simulink model "RPBC5602016"  (R2016b)
settings: Solver=ode45  StartTime=0.0  StopTime=100  RelTol=1e-3  EnableMultiTasking=on
values from neighbouring files (symbols this model uses):
  A1 = 1    [setupRPBC.m]
  A2 = 0.25    [setupRPBC.m]
  A3 = 0.5    [setupRPBC.m]
  A_Matrix = [A_Matrix a]    [systemident.m]
  alpha = mean(alpha)    [systemident.m]
  b1 = 0    [setupRPBC.m]
  b2 = 0    [setupRPBC.m]
  b3 = -pi/2    (= -1.57079632679)    [setupRPBC.m]
  B_Matrix = [B_Matrix B_e]    [systemident.m]
  C = 10    [RUN.m]
  N =     [Gear Ratios.mat]
  R = mean(R)    [systemident.m]
  w1 = 2    [setupRPBC.m]
  w2 = 2    [setupRPBC.m]
  w3 = 2    [setupRPBC.m]
  Z0 = [0;0;0;0;-pi/2;0]    [setupRPBC.m]
undefined symbols (not defined in the file or in its folder): statederPUMA3
settings Model: ExtModeAutoUpdateStatusClock=off  Creator=rhanz  LastModifiedBy=R4hul
settings DataIOCC: LimitDataPoints=on  SaveFormat=Array  SignalLoggingSaveFormat=ModelDataLogs
settings OptimizationCC: ExpressionDepthLimit=2147483647  InitFltsAndDblsToZero=on  LifeSpan=inf
settings DebuggingCC: SaveWithParameterizedLinksMsg=none  UnderspecifiedInitializationDetection=Classic  MergeDetectMultiDrivingBlocksExec=none  SignalResolutionControl=TryResolveAllWithWarning  MultiTaskDSMMsg=warning  MultiTaskCondExecSysMsg=none  FcnCallInpInsideContextMsg=warning  StateNameClashWarn=warning  SFUnexpectedBacktrackingDiag=warning  SFNoUnconditionalDefaultTransitionDiag=warning  SFExecutionAtInitializationDiag=none
settings HardwareCC: ProdBitPerPointer=32  ProdBitPerSizeT=32  ProdBitPerPtrDiffT=32  ProdLargestAtomicFloat=None  ProdIntDivRoundTo=Undefined  ProdEndianess=Unspecified  ProdWordSize=32  ProdHWDeviceType=32-bit Generic
settings ModelReferenceCC: PropagateSignalLabelsOutOfModel=off
settings GRTTargetCC: TargetFcnLib=ansi_tfl_tmw.mat  TargetLangStandard=C89/C90 (ANSI)  GeneratePreprocessorConditionals=Disable all  CombineOutputUpdateFcns=off  GRTInterface=on
settings ConfigComp: CovMetricSettings=dw  CovHtmlReporting=on  CovSaveCumulativeToWorkspaceVar=on  CovSaveSingleToWorkspaceVar=on  CovExternalEMLEnable=off

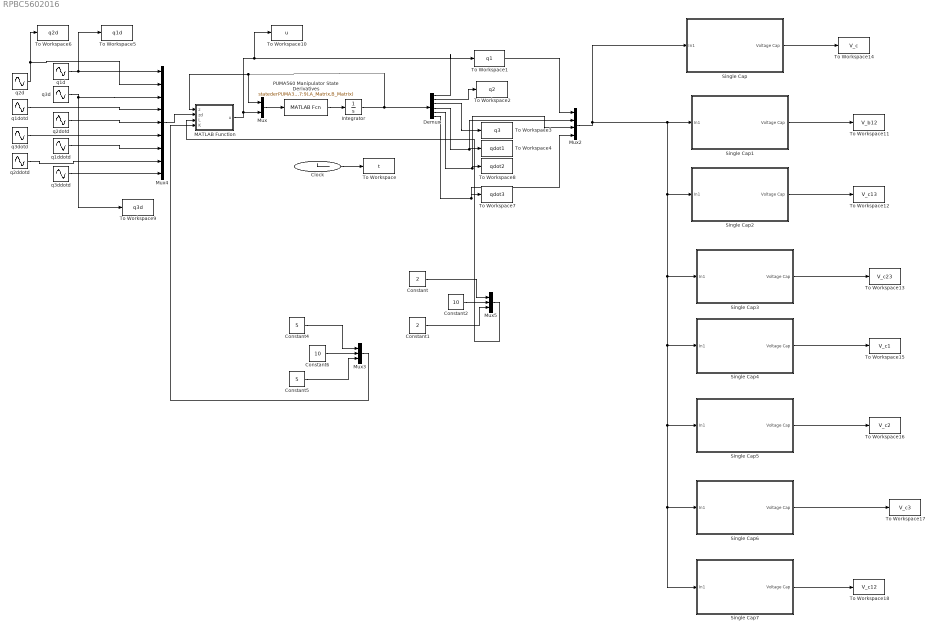
== system RPBC5602016 ==
  Clock : Clock
  Constant : Constant  Value=2
  Constant1 : Constant  Value=2
  Constant2 : Constant  Value=10
  Constant4 : Constant  Value=5
  Constant5 : Constant  Value=5
  Constant6 : Constant  Value=10
  Demux : Demux  Outputs=6
  Integrator : Integrator  InitialCondition=Z0
  MATLAB Function : MATLAB Function  TreatAsAtomicUnit=on
  Mux : Mux  Inputs=2
  Mux2 : Mux
  Mux3 : Mux  Inputs=3
  Mux4 : Mux  Inputs=9
  Mux5 : Mux  Inputs=3
  PUMA560 Manipulator State Derivatives : MATLABFcn  MATLABFcn=statederPUMA3(u(1:6),u(7:9),A_Matrix,B_Matrix)  OutputDimensions=6
  Single Cap : Subsystem
  Single Cap1 : Subsystem
  Single Cap2 : Subsystem
  Single Cap3 : Subsystem
  Single Cap4 : Subsystem
  Single Cap5 : Subsystem
  Single Cap6 : Subsystem
  Single Cap7 : Subsystem
  To Workspace : ToWorkspace  VariableName=t  SampleTime=-1
  To Workspace1 : ToWorkspace  VariableName=q1  SampleTime=-1
  To Workspace10 : ToWorkspace  VariableName=u  SampleTime=-1
  To Workspace11 : ToWorkspace  VariableName=V_b12  SampleTime=-1
  To Workspace12 : ToWorkspace  VariableName=V_c13  SampleTime=-1
  To Workspace13 : ToWorkspace  VariableName=V_c23  SampleTime=-1
  To Workspace14 : ToWorkspace  VariableName=V_c  SampleTime=-1
  To Workspace15 : ToWorkspace  VariableName=V_c1  SampleTime=-1
  To Workspace16 : ToWorkspace  VariableName=V_c2  SampleTime=-1
  To Workspace17 : ToWorkspace  VariableName=V_c3  SampleTime=-1
  To Workspace18 : ToWorkspace  VariableName=V_c12  SampleTime=-1
  To Workspace2 : ToWorkspace  VariableName=q2  SampleTime=-1
  To Workspace3 : ToWorkspace  VariableName=q3  SampleTime=-1
  To Workspace4 : ToWorkspace  VariableName=qdot1  SampleTime=-1
  To Workspace5 : ToWorkspace  VariableName=q1d  SampleTime=-1
  To Workspace6 : ToWorkspace  VariableName=q2d  SampleTime=-1
  To Workspace7 : ToWorkspace  VariableName=qdot3  SampleTime=-1
  To Workspace8 : ToWorkspace  VariableName=qdot2  SampleTime=-1
  To Workspace9 : ToWorkspace  VariableName=q3d  SampleTime=-1
  q1d : Sin  Amplitude=A1  Bias=b1  Frequency=w1  SampleTime=0
  q1ddotd : Sin  Amplitude=A1*w1^2  Frequency=w1  Phase=pi  SampleTime=0
  q1dotd : Sin  Amplitude=A1*w1  Frequency=w1  Phase=pi/2  SampleTime=0
  q2d : Sin  Amplitude=A2  Bias=b2  Frequency=w2  SampleTime=0
  q2ddotd : Sin  Amplitude=A2*w2^2  Frequency=w2  Phase=pi  SampleTime=0
  q2dotd : Sin  Amplitude=A2*w2  Frequency=w2  Phase=pi/2  SampleTime=0
  q3d : Sin  Amplitude=A3  Bias=b3  Frequency=w3  SampleTime=0
  q3ddotd : Sin  Amplitude=A3*w3^2  Frequency=w3  Phase=pi  SampleTime=0
  q3dotd : Sin  Amplitude=A3*w3  Frequency=w3  Phase=pi/2  SampleTime=0
  wires:
  PUMA560 Manipulator State Derivatives/1 -> Integrator/1
  Integrator/1 -> MATLAB Function/1(z), Mux/1, Demux/1
  Mux/1 -> PUMA560 Manipulator State Derivatives/1
  Clock/1 -> To Workspace/1
  Demux/1 -> To Workspace1/1
  Demux/3 -> To Workspace3/1
  Demux/4 -> Mux2/2, To Workspace4/1
  q1d/1 -> Mux4/1, To Workspace5/1
  q2d/1 -> Mux4/2, To Workspace6/1
  q3d/1 -> Mux4/3, To Workspace9/1
  Demux/2 -> To Workspace2/1
  Demux/5 -> Mux2/3, To Workspace8/1
  Demux/6 -> Mux2/4, To Workspace7/1
  MATLAB Function/1(u) -> Mux2/1, To Workspace10/1, Mux/2
  Single Cap/1(Voltage Cap) -> To Workspace14/1
  Mux2/1 -> Single Cap7/1(In1), Single Cap6/1(In1), Single Cap5/1(In1), Single Cap4/1(In1), Single Cap3/1(In1), Single Cap2/1(In1), Single Cap1/1(In1), Single Cap/1(In1)
  Single Cap1/1(Voltage Cap) -> To Workspace11/1
  Single Cap2/1(Voltage Cap) -> To Workspace12/1
  Single Cap3/1(Voltage Cap) -> To Workspace13/1
  Single Cap4/1(Voltage Cap) -> To Workspace15/1
  Single Cap6/1(Voltage Cap) -> To Workspace17/1
  Single Cap5/1(Voltage Cap) -> To Workspace16/1
  Single Cap7/1(Voltage Cap) -> To Workspace18/1
  Constant5/1 -> Mux3/3
  Constant6/1 -> Mux3/2
  Constant4/1 -> Mux3/1
  Mux3/1 -> MATLAB Function/4(K)
  Constant2/1 -> Mux5/2
  Constant1/1 -> Mux5/3
  Constant/1 -> Mux5/1
  Mux5/1 -> MATLAB Function/3(L)
  Mux4/1 -> MATLAB Function/2(zd)
  q1dotd/1 -> Mux4/4
  q2dotd/1 -> Mux4/5
  q3dotd/1 -> Mux4/6
  q1ddotd/1 -> Mux4/7
  q2ddotd/1 -> Mux4/8
  q3ddotd/1 -> Mux4/9

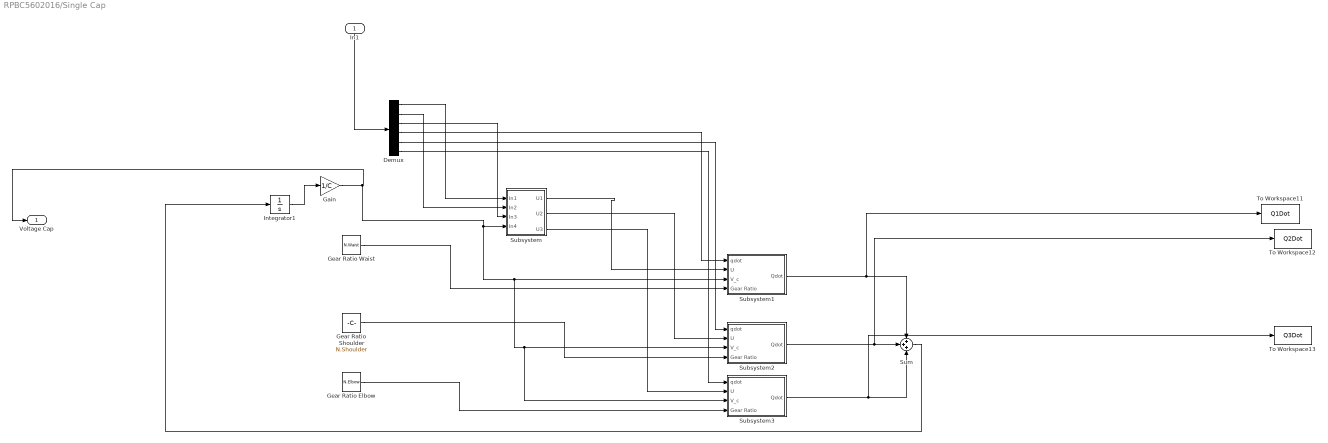
== system RPBC5602016/Single Cap ==
  In1 : Inport
  Demux : Demux  Outputs=6
  Gain : Gain  Gain=1/C
  Gear Ratio Elbow : Constant  Value=N.Elbow
  "Gear Ratio Shoulder " : Constant  Value=N.Shoulder
  Gear Ratio Waist : Constant  Value=N.Waist
  Integrator1 : Integrator  InitialCondition=C*30
  Subsystem : Subsystem
  Subsystem1 : Subsystem
  Subsystem2 : Subsystem
  Subsystem3 : Subsystem
  Sum : Sum  Inputs=3
  To Workspace11 : ToWorkspace  VariableName=Q1Dot  SampleTime=-1
  To Workspace12 : ToWorkspace  VariableName=Q2Dot  SampleTime=-1
  To Workspace13 : ToWorkspace  VariableName=Q3Dot  SampleTime=-1
  Voltage Cap : Outport
  wires:
  Subsystem/2(U2) -> Subsystem2/2(U)
  Gear Ratio Waist/1 -> Subsystem1/4(Gear Ratio)
  Subsystem/1(U1) -> Subsystem1/2(U)
  Subsystem3/1(Qdot) -> To Workspace13/1, Sum/3
  Integrator1/1 -> Gain/1
  Subsystem1/1(Qdot) -> To Workspace11/1, Sum/1
  Subsystem/3(U3) -> Subsystem3/2(U)
  Subsystem2/1(Qdot) -> To Workspace12/1, Sum/2
  Sum/1 -> Integrator1/1
  Gear Ratio Elbow/1 -> Subsystem3/4(Gear Ratio)
  "Gear Ratio Shoulder "/1 -> Subsystem2/4(Gear Ratio)
  Gain/1 -> Subsystem/4(In4), Subsystem3/3(V_c), Subsystem2/3(V_c), Subsystem1/3(V_c), Voltage Cap/1
  In1/1 -> Demux/1
  Demux/1 -> Subsystem/1(In1)
  Demux/2 -> Subsystem/2(In2)
  Demux/3 -> Subsystem/3(In3)
  Demux/4 -> Subsystem1/1(qdot)
  Demux/5 -> Subsystem2/1(qdot)
  Demux/6 -> Subsystem3/1(qdot)

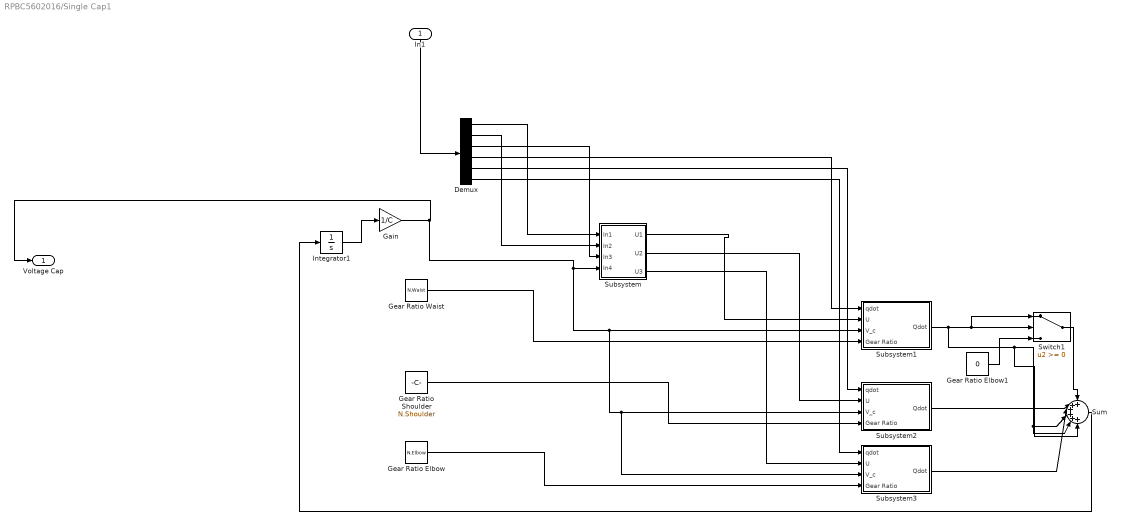
== system RPBC5602016/Single Cap1 ==
  In1 : Inport
  Demux : Demux  Outputs=6
  Gain : Gain  Gain=1/C
  Gear Ratio Elbow : Constant  Value=N.Elbow
  Gear Ratio Elbow1 : Constant  Value=0
  "Gear Ratio Shoulder " : Constant  Value=N.Shoulder
  Gear Ratio Waist : Constant  Value=N.Waist
  Integrator1 : Integrator  InitialCondition=C*30
  Subsystem : Subsystem
  Subsystem1 : Subsystem
  Subsystem2 : Subsystem
  Subsystem3 : Subsystem
  Sum : Sum  Inputs=6
  Switch1 : Switch
  Voltage Cap : Outport
  wires:
  Demux/6 -> Subsystem3/1(qdot)
  Demux/5 -> Subsystem2/1(qdot)
  Demux/4 -> Subsystem1/1(qdot)
  Demux/3 -> Subsystem/3(In3)
  Demux/2 -> Subsystem/2(In2)
  Demux/1 -> Subsystem/1(In1)
  In1/1 -> Demux/1
  Gain/1 -> Voltage Cap/1, Subsystem1/3(V_c), Subsystem2/3(V_c), Subsystem3/3(V_c), Subsystem/4(In4)
  "Gear Ratio Shoulder "/1 -> Subsystem2/4(Gear Ratio)
  Gear Ratio Elbow/1 -> Subsystem3/4(Gear Ratio)
  Subsystem2/1(Qdot) -> Sum/2
  Subsystem/3(U3) -> Subsystem3/2(U)
  Integrator1/1 -> Gain/1
  Subsystem/1(U1) -> Subsystem1/2(U)
  Gear Ratio Waist/1 -> Subsystem1/4(Gear Ratio)
  Subsystem/2(U2) -> Subsystem2/2(U)
  Subsystem3/1(Qdot) -> Sum/3
  Sum/1 -> Integrator1/1
  Subsystem1/1(Qdot) -> Sum/6, Sum/5, Sum/4, Switch1/1, Switch1/2
  Switch1/1 -> Sum/1
  Gear Ratio Elbow1/1 -> Switch1/3

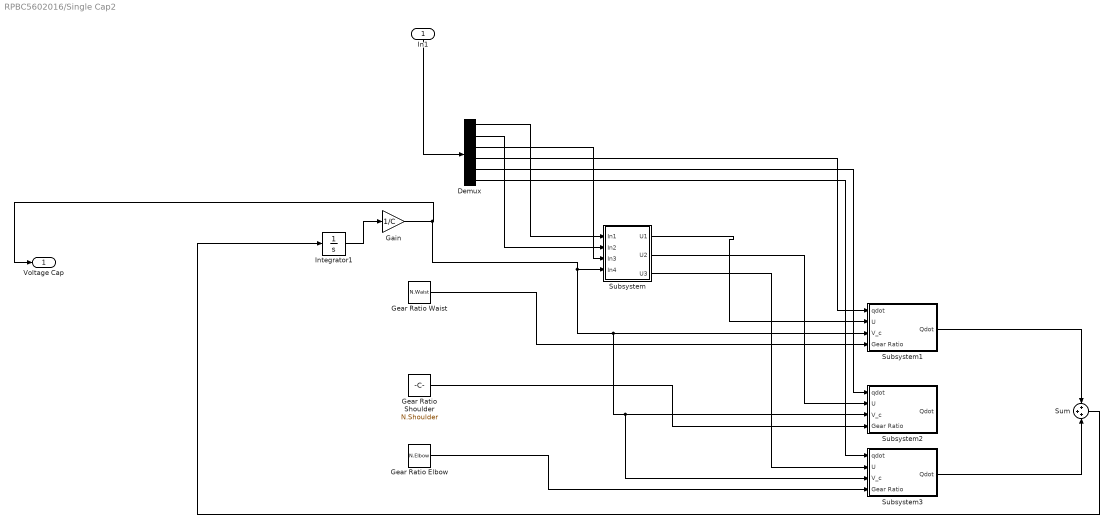
== system RPBC5602016/Single Cap2 ==
  In1 : Inport
  Demux : Demux  Outputs=6
  Gain : Gain  Gain=1/C
  Gear Ratio Elbow : Constant  Value=N.Elbow
  "Gear Ratio Shoulder " : Constant  Value=N.Shoulder
  Gear Ratio Waist : Constant  Value=N.Waist
  Integrator1 : Integrator  InitialCondition=C*30
  Subsystem : Subsystem
  Subsystem1 : Subsystem
  Subsystem2 : Subsystem
  Subsystem3 : Subsystem
  Sum : Sum  Inputs=3
  Voltage Cap : Outport
  wires:
  Subsystem/2(U2) -> Subsystem2/2(U)
  Gear Ratio Waist/1 -> Subsystem1/4(Gear Ratio)
  Subsystem/1(U1) -> Subsystem1/2(U)
  Subsystem3/1(Qdot) -> Sum/3
  Integrator1/1 -> Gain/1
  Subsystem1/1(Qdot) -> Sum/1
  Subsystem/3(U3) -> Subsystem3/2(U)
  Sum/1 -> Integrator1/1
  Gear Ratio Elbow/1 -> Subsystem3/4(Gear Ratio)
  "Gear Ratio Shoulder "/1 -> Subsystem2/4(Gear Ratio)
  Gain/1 -> Subsystem/4(In4), Subsystem3/3(V_c), Subsystem2/3(V_c), Subsystem1/3(V_c), Voltage Cap/1
  In1/1 -> Demux/1
  Demux/1 -> Subsystem/1(In1)
  Demux/2 -> Subsystem/2(In2)
  Demux/3 -> Subsystem/3(In3)
  Demux/4 -> Subsystem1/1(qdot)
  Demux/5 -> Subsystem2/1(qdot)
  Demux/6 -> Subsystem3/1(qdot)

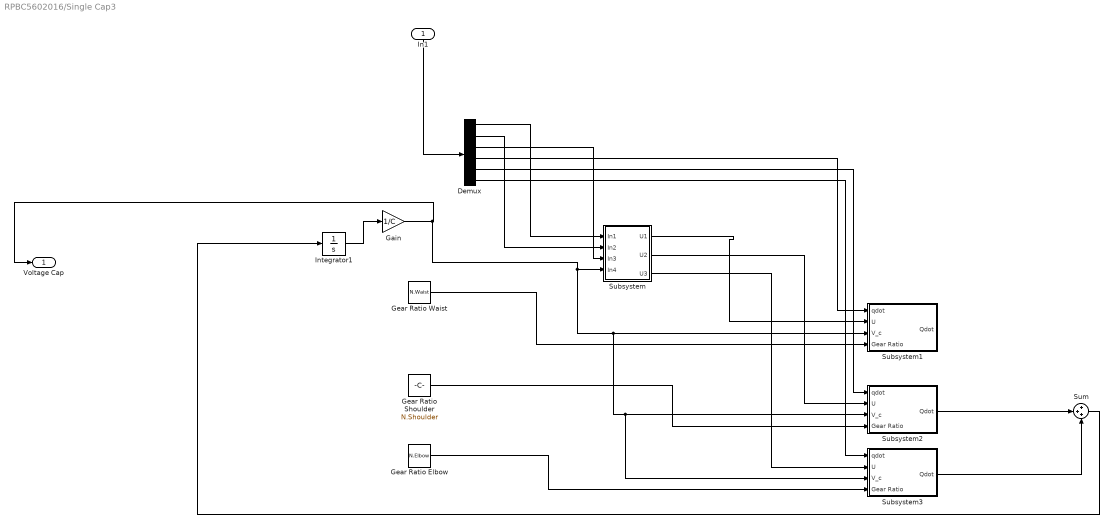
== system RPBC5602016/Single Cap3 ==
  In1 : Inport
  Demux : Demux  Outputs=6
  Gain : Gain  Gain=1/C
  Gear Ratio Elbow : Constant  Value=N.Elbow
  "Gear Ratio Shoulder " : Constant  Value=N.Shoulder
  Gear Ratio Waist : Constant  Value=N.Waist
  Integrator1 : Integrator  InitialCondition=C*30
  Subsystem : Subsystem
  Subsystem1 : Subsystem
  Subsystem2 : Subsystem
  Subsystem3 : Subsystem
  Sum : Sum  Inputs=3
  Voltage Cap : Outport
  wires:
  Demux/6 -> Subsystem3/1(qdot)
  Demux/5 -> Subsystem2/1(qdot)
  Demux/4 -> Subsystem1/1(qdot)
  Demux/3 -> Subsystem/3(In3)
  Demux/2 -> Subsystem/2(In2)
  Demux/1 -> Subsystem/1(In1)
  In1/1 -> Demux/1
  Gain/1 -> Voltage Cap/1, Subsystem1/3(V_c), Subsystem2/3(V_c), Subsystem3/3(V_c), Subsystem/4(In4)
  "Gear Ratio Shoulder "/1 -> Subsystem2/4(Gear Ratio)
  Gear Ratio Elbow/1 -> Subsystem3/4(Gear Ratio)
  Sum/1 -> Integrator1/1
  Subsystem2/1(Qdot) -> Sum/2
  Subsystem/3(U3) -> Subsystem3/2(U)
  Integrator1/1 -> Gain/1
  Subsystem3/1(Qdot) -> Sum/3
  Subsystem/1(U1) -> Subsystem1/2(U)
  Gear Ratio Waist/1 -> Subsystem1/4(Gear Ratio)
  Subsystem/2(U2) -> Subsystem2/2(U)

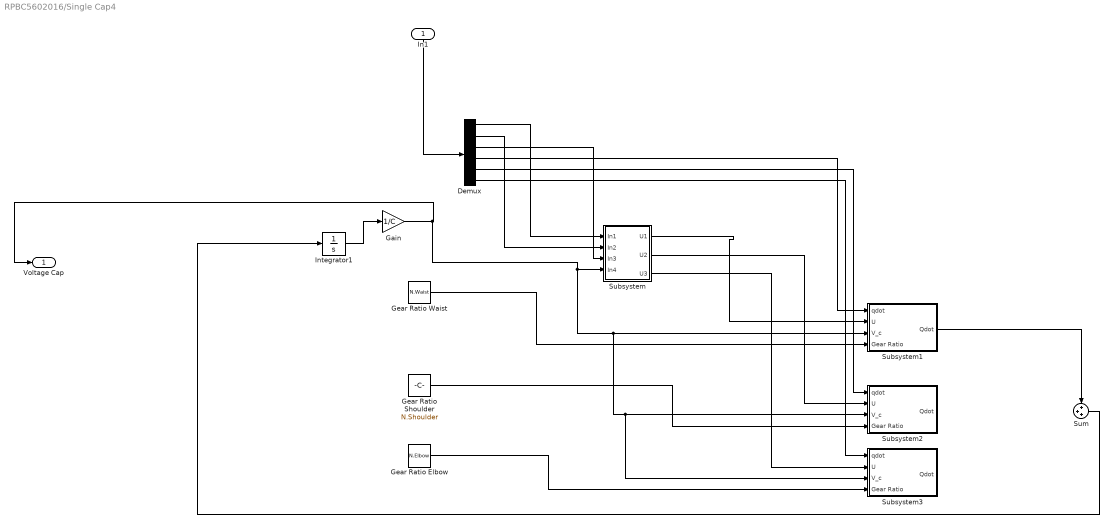
== system RPBC5602016/Single Cap4 ==
  In1 : Inport
  Demux : Demux  Outputs=6
  Gain : Gain  Gain=1/C
  Gear Ratio Elbow : Constant  Value=N.Elbow
  "Gear Ratio Shoulder " : Constant  Value=N.Shoulder
  Gear Ratio Waist : Constant  Value=N.Waist
  Integrator1 : Integrator  InitialCondition=C*30
  Subsystem : Subsystem
  Subsystem1 : Subsystem
  Subsystem2 : Subsystem
  Subsystem3 : Subsystem
  Sum : Sum  Inputs=3
  Voltage Cap : Outport
  wires:
  Subsystem/2(U2) -> Subsystem2/2(U)
  Gear Ratio Waist/1 -> Subsystem1/4(Gear Ratio)
  Subsystem/1(U1) -> Subsystem1/2(U)
  Integrator1/1 -> Gain/1
  Subsystem/3(U3) -> Subsystem3/2(U)
  Sum/1 -> Integrator1/1
  Gear Ratio Elbow/1 -> Subsystem3/4(Gear Ratio)
  "Gear Ratio Shoulder "/1 -> Subsystem2/4(Gear Ratio)
  Gain/1 -> Subsystem/4(In4), Subsystem3/3(V_c), Subsystem2/3(V_c), Subsystem1/3(V_c), Voltage Cap/1
  In1/1 -> Demux/1
  Demux/1 -> Subsystem/1(In1)
  Demux/2 -> Subsystem/2(In2)
  Demux/3 -> Subsystem/3(In3)
  Demux/4 -> Subsystem1/1(qdot)
  Demux/5 -> Subsystem2/1(qdot)
  Demux/6 -> Subsystem3/1(qdot)
  Subsystem1/1(Qdot) -> Sum/1

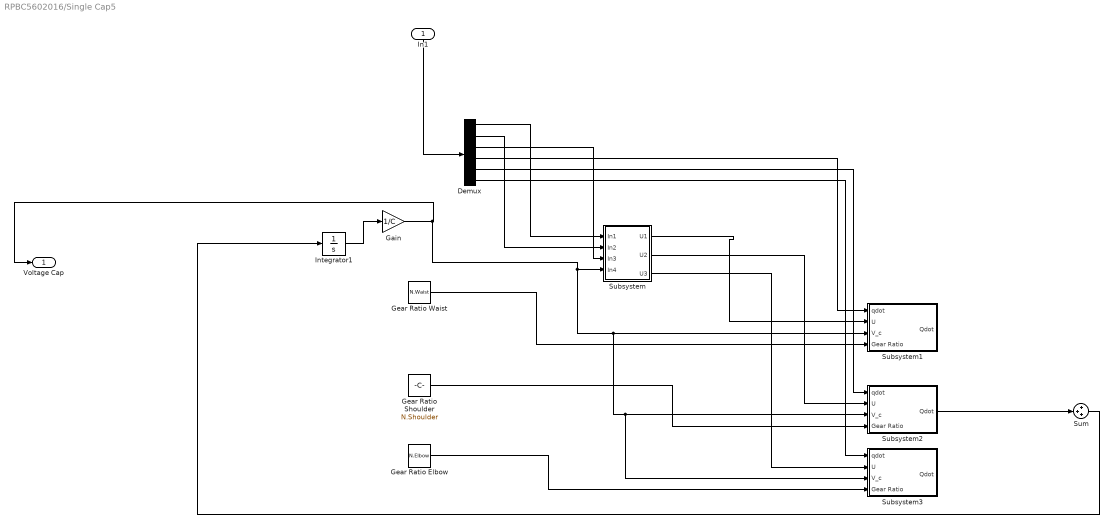
== system RPBC5602016/Single Cap5 ==
  In1 : Inport
  Demux : Demux  Outputs=6
  Gain : Gain  Gain=1/C
  Gear Ratio Elbow : Constant  Value=N.Elbow
  "Gear Ratio Shoulder " : Constant  Value=N.Shoulder
  Gear Ratio Waist : Constant  Value=N.Waist
  Integrator1 : Integrator  InitialCondition=C*30
  Subsystem : Subsystem
  Subsystem1 : Subsystem
  Subsystem2 : Subsystem
  Subsystem3 : Subsystem
  Sum : Sum  Inputs=3
  Voltage Cap : Outport
  wires:
  Demux/6 -> Subsystem3/1(qdot)
  Demux/5 -> Subsystem2/1(qdot)
  Demux/4 -> Subsystem1/1(qdot)
  Demux/3 -> Subsystem/3(In3)
  Demux/2 -> Subsystem/2(In2)
  Demux/1 -> Subsystem/1(In1)
  In1/1 -> Demux/1
  Gain/1 -> Voltage Cap/1, Subsystem1/3(V_c), Subsystem2/3(V_c), Subsystem3/3(V_c), Subsystem/4(In4)
  "Gear Ratio Shoulder "/1 -> Subsystem2/4(Gear Ratio)
  Gear Ratio Elbow/1 -> Subsystem3/4(Gear Ratio)
  Sum/1 -> Integrator1/1
  Subsystem2/1(Qdot) -> Sum/2
  Subsystem/3(U3) -> Subsystem3/2(U)
  Integrator1/1 -> Gain/1
  Subsystem/1(U1) -> Subsystem1/2(U)
  Gear Ratio Waist/1 -> Subsystem1/4(Gear Ratio)
  Subsystem/2(U2) -> Subsystem2/2(U)

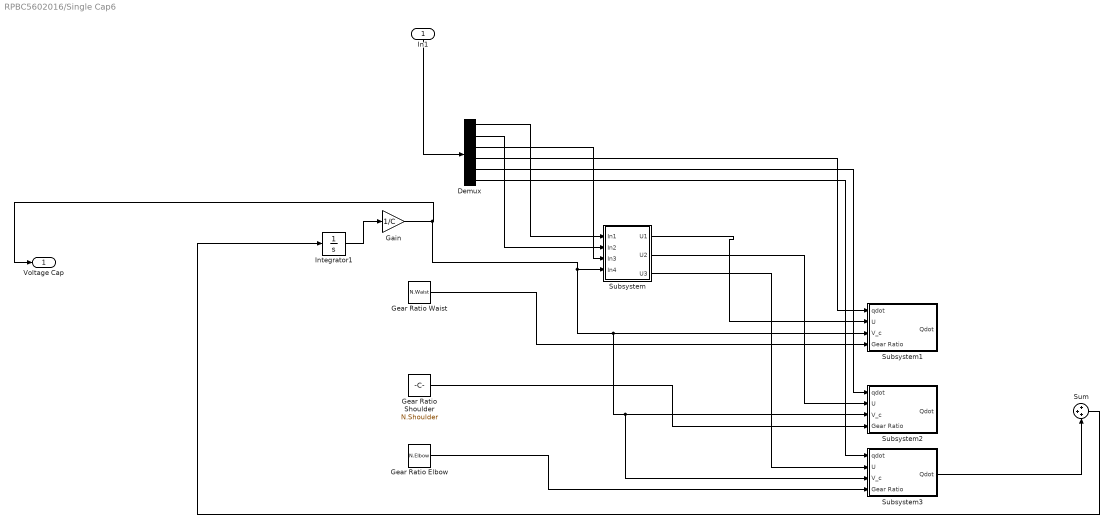
== system RPBC5602016/Single Cap6 ==
  In1 : Inport
  Demux : Demux  Outputs=6
  Gain : Gain  Gain=1/C
  Gear Ratio Elbow : Constant  Value=N.Elbow
  "Gear Ratio Shoulder " : Constant  Value=N.Shoulder
  Gear Ratio Waist : Constant  Value=N.Waist
  Integrator1 : Integrator  InitialCondition=C*30
  Subsystem : Subsystem
  Subsystem1 : Subsystem
  Subsystem2 : Subsystem
  Subsystem3 : Subsystem
  Sum : Sum  Inputs=3
  Voltage Cap : Outport
  wires:
  Subsystem/2(U2) -> Subsystem2/2(U)
  Gear Ratio Waist/1 -> Subsystem1/4(Gear Ratio)
  Subsystem/1(U1) -> Subsystem1/2(U)
  Subsystem3/1(Qdot) -> Sum/3
  Integrator1/1 -> Gain/1
  Subsystem/3(U3) -> Subsystem3/2(U)
  Sum/1 -> Integrator1/1
  Gear Ratio Elbow/1 -> Subsystem3/4(Gear Ratio)
  "Gear Ratio Shoulder "/1 -> Subsystem2/4(Gear Ratio)
  Gain/1 -> Subsystem/4(In4), Subsystem3/3(V_c), Subsystem2/3(V_c), Subsystem1/3(V_c), Voltage Cap/1
  In1/1 -> Demux/1
  Demux/1 -> Subsystem/1(In1)
  Demux/2 -> Subsystem/2(In2)
  Demux/3 -> Subsystem/3(In3)
  Demux/4 -> Subsystem1/1(qdot)
  Demux/5 -> Subsystem2/1(qdot)
  Demux/6 -> Subsystem3/1(qdot)

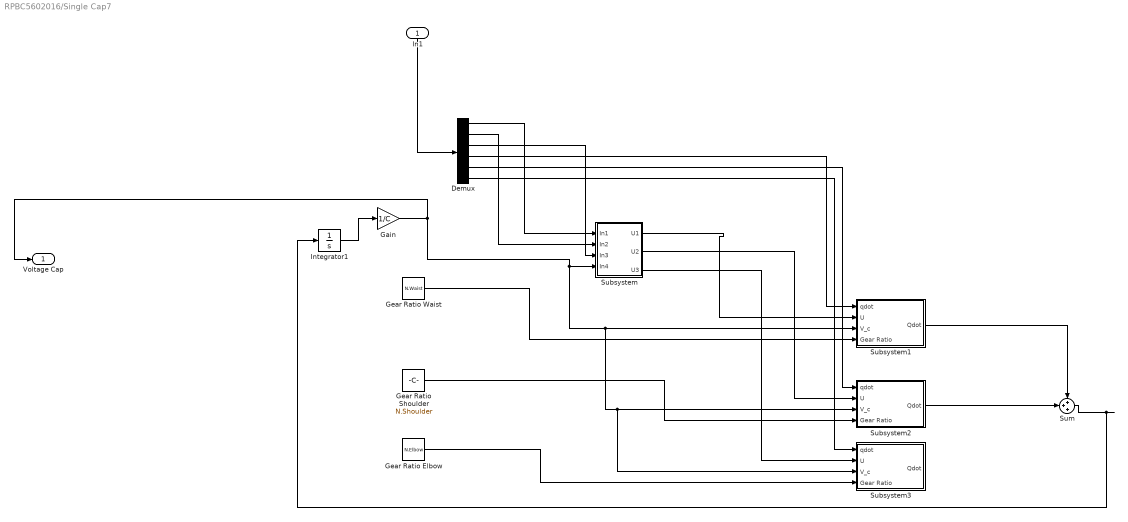
== system RPBC5602016/Single Cap7 ==
  In1 : Inport
  Demux : Demux  Outputs=6
  Gain : Gain  Gain=1/C
  Gear Ratio Elbow : Constant  Value=N.Elbow
  "Gear Ratio Shoulder " : Constant  Value=N.Shoulder
  Gear Ratio Waist : Constant  Value=N.Waist
  Integrator1 : Integrator  InitialCondition=C*30
  Subsystem : Subsystem
  Subsystem1 : Subsystem
  Subsystem2 : Subsystem
  Subsystem3 : Subsystem
  Sum : Sum  Inputs=3
  Voltage Cap : Outport
  wires:
  Sum/1 -> Integrator1/1
  Subsystem/2(U2) -> Subsystem2/2(U)
  Gear Ratio Waist/1 -> Subsystem1/4(Gear Ratio)
  Subsystem/1(U1) -> Subsystem1/2(U)
  Integrator1/1 -> Gain/1
  Subsystem1/1(Qdot) -> Sum/1
  Subsystem/3(U3) -> Subsystem3/2(U)
  Subsystem2/1(Qdot) -> Sum/2
  Gear Ratio Elbow/1 -> Subsystem3/4(Gear Ratio)
  "Gear Ratio Shoulder "/1 -> Subsystem2/4(Gear Ratio)
  Gain/1 -> Subsystem/4(In4), Subsystem3/3(V_c), Subsystem2/3(V_c), Subsystem1/3(V_c), Voltage Cap/1
  In1/1 -> Demux/1
  Demux/1 -> Subsystem/1(In1)
  Demux/2 -> Subsystem/2(In2)
  Demux/3 -> Subsystem/3(In3)
  Demux/4 -> Subsystem1/1(qdot)
  Demux/5 -> Subsystem2/1(qdot)
  Demux/6 -> Subsystem3/1(qdot)

== system RPBC5602016/Single Cap/Subsystem ==
  In1 : Inport
  In2 : Inport  Port=2
  In3 : Inport  Port=3
  In4 : Inport  Port=4
  Divide : Product  Inputs=*/
  Divide1 : Product  Inputs=*/
  Divide2 : Product  Inputs=*/
  U1 : Outport
  U2 : Outport  Port=2
  U3 : Outport  Port=3
  wires:
  Divide2/1 -> U3/1
  Divide1/1 -> U2/1
  Divide/1 -> U1/1
  In1/1 -> Divide/1
  In2/1 -> Divide1/1
  In3/1 -> Divide2/1
  In4/1 -> Divide2/2, Divide1/2, Divide/2

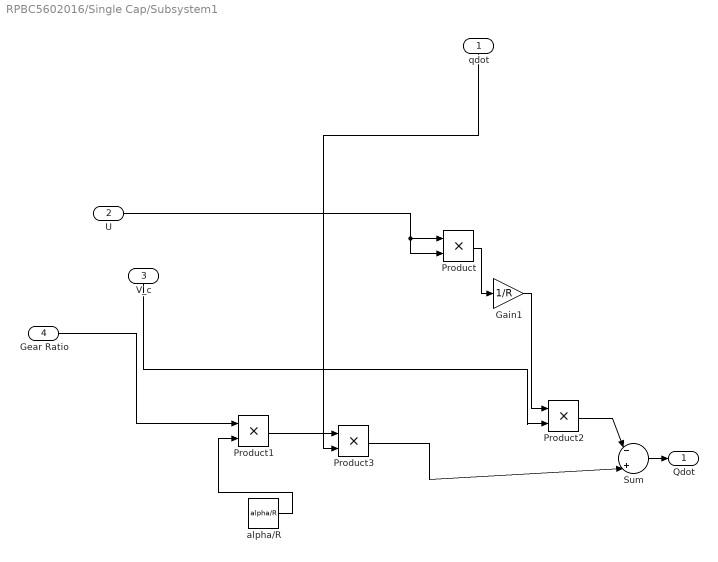
== system RPBC5602016/Single Cap/Subsystem1 ==
  qdot : Inport
  U : Inport  Port=2
  V_c : Inport  Port=3
  Gear Ratio : Inport  Port=4
  Gain1 : Gain  Gain=1/R
  Product{,1..3} (4 alike) : Product
  Sum : Sum  Inputs=|-|+|
  alpha/R : Constant  Value=alpha/R
  Qdot : Outport
  wires:
  Product2/1 -> Sum/1
  qdot/1 -> Product3/2
  V_c/1 -> Product2/2
  Sum/1 -> Qdot/1
  alpha/R/1 -> Product1/2
  Product/1 -> Gain1/1
  U/1 -> Product/2, Product/1
  Product3/1 -> Sum/2
  Product1/1 -> Product3/1
  Gain1/1 -> Product2/1
  Gear Ratio/1 -> Product1/1

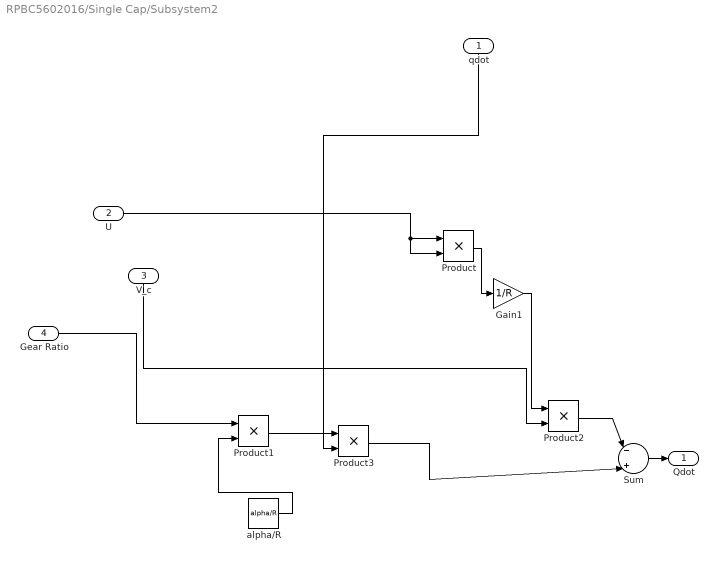
== system RPBC5602016/Single Cap/Subsystem2 ==
  qdot : Inport
  U : Inport  Port=2
  V_c : Inport  Port=3
  Gear Ratio : Inport  Port=4
  Gain1 : Gain  Gain=1/R
  Product{,1..3} (4 alike) : Product
  Sum : Sum  Inputs=|-|+|
  alpha/R : Constant  Value=alpha/R
  Qdot : Outport
  wires:
  Gear Ratio/1 -> Product1/1
  Gain1/1 -> Product2/1
  Product1/1 -> Product3/1
  Product3/1 -> Sum/2
  U/1 -> Product/1, Product/2
  Product/1 -> Gain1/1
  alpha/R/1 -> Product1/2
  Sum/1 -> Qdot/1
  V_c/1 -> Product2/2
  qdot/1 -> Product3/2
  Product2/1 -> Sum/1

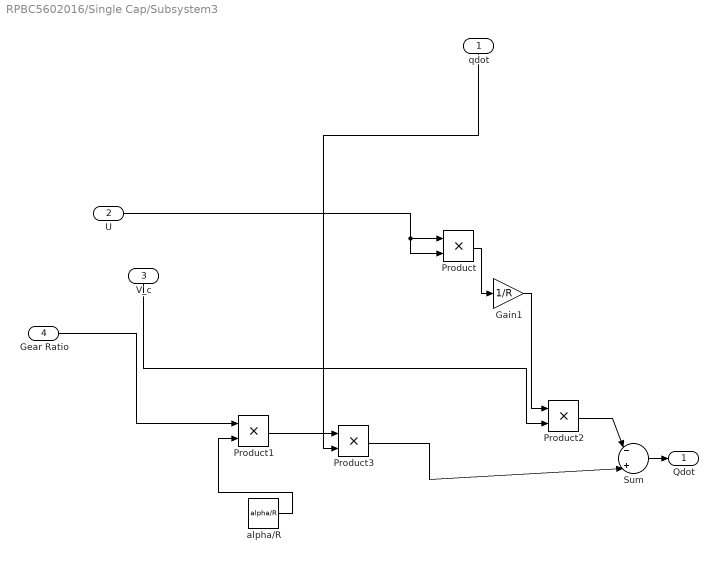
== system RPBC5602016/Single Cap/Subsystem3 ==
  qdot : Inport
  U : Inport  Port=2
  V_c : Inport  Port=3
  Gear Ratio : Inport  Port=4
  Gain1 : Gain  Gain=1/R
  Product{,1..3} (4 alike) : Product
  Sum : Sum  Inputs=|-|+|
  alpha/R : Constant  Value=alpha/R
  Qdot : Outport
  wires:
  Product2/1 -> Sum/1
  qdot/1 -> Product3/2
  V_c/1 -> Product2/2
  Sum/1 -> Qdot/1
  alpha/R/1 -> Product1/2
  Product/1 -> Gain1/1
  U/1 -> Product/2, Product/1
  Product3/1 -> Sum/2
  Product1/1 -> Product3/1
  Gain1/1 -> Product2/1
  Gear Ratio/1 -> Product1/1

== system RPBC5602016/Single Cap1/Subsystem ==
  In1 : Inport
  In2 : Inport  Port=2
  In3 : Inport  Port=3
  In4 : Inport  Port=4
  Divide : Product  Inputs=*/
  Divide1 : Product  Inputs=*/
  Divide2 : Product  Inputs=*/
  U1 : Outport
  U2 : Outport  Port=2
  U3 : Outport  Port=3
  wires:
  In4/1 -> Divide/2, Divide1/2, Divide2/2
  In3/1 -> Divide2/1
  In2/1 -> Divide1/1
  In1/1 -> Divide/1
  Divide/1 -> U1/1
  Divide1/1 -> U2/1
  Divide2/1 -> U3/1

== system RPBC5602016/Single Cap1/Subsystem1 ==
  qdot : Inport
  U : Inport  Port=2
  V_c : Inport  Port=3
  Gear Ratio : Inport  Port=4
  Gain1 : Gain  Gain=1/R
  Product{,1..3} (4 alike) : Product
  Sum : Sum  Inputs=|-|+|
  alpha/R : Constant  Value=alpha/R
  Qdot : Outport
  wires:
  Gear Ratio/1 -> Product1/1
  Gain1/1 -> Product2/1
  Product1/1 -> Product3/1
  Product3/1 -> Sum/2
  U/1 -> Product/1, Product/2
  Product/1 -> Gain1/1
  alpha/R/1 -> Product1/2
  Sum/1 -> Qdot/1
  V_c/1 -> Product2/2
  qdot/1 -> Product3/2
  Product2/1 -> Sum/1

== system RPBC5602016/Single Cap1/Subsystem2 ==
  qdot : Inport
  U : Inport  Port=2
  V_c : Inport  Port=3
  Gear Ratio : Inport  Port=4
  Gain1 : Gain  Gain=1/R
  Product{,1..3} (4 alike) : Product
  Sum : Sum  Inputs=|-|+|
  alpha/R : Constant  Value=alpha/R
  Qdot : Outport
  wires:
  Product2/1 -> Sum/1
  qdot/1 -> Product3/2
  V_c/1 -> Product2/2
  Sum/1 -> Qdot/1
  alpha/R/1 -> Product1/2
  Product/1 -> Gain1/1
  U/1 -> Product/2, Product/1
  Product3/1 -> Sum/2
  Product1/1 -> Product3/1
  Gain1/1 -> Product2/1
  Gear Ratio/1 -> Product1/1

== system RPBC5602016/Single Cap1/Subsystem3 ==
  qdot : Inport
  U : Inport  Port=2
  V_c : Inport  Port=3
  Gear Ratio : Inport  Port=4
  Gain1 : Gain  Gain=1/R
  Product{,1..3} (4 alike) : Product
  Sum : Sum  Inputs=|-|+|
  alpha/R : Constant  Value=alpha/R
  Qdot : Outport
  wires:
  Gear Ratio/1 -> Product1/1
  Gain1/1 -> Product2/1
  Product1/1 -> Product3/1
  Product3/1 -> Sum/2
  U/1 -> Product/1, Product/2
  Product/1 -> Gain1/1
  alpha/R/1 -> Product1/2
  Sum/1 -> Qdot/1
  V_c/1 -> Product2/2
  qdot/1 -> Product3/2
  Product2/1 -> Sum/1

== system RPBC5602016/Single Cap2/Subsystem ==
  In1 : Inport
  In2 : Inport  Port=2
  In3 : Inport  Port=3
  In4 : Inport  Port=4
  Divide : Product  Inputs=*/
  Divide1 : Product  Inputs=*/
  Divide2 : Product  Inputs=*/
  U1 : Outport
  U2 : Outport  Port=2
  U3 : Outport  Port=3
  wires:
  Divide2/1 -> U3/1
  Divide1/1 -> U2/1
  Divide/1 -> U1/1
  In1/1 -> Divide/1
  In2/1 -> Divide1/1
  In3/1 -> Divide2/1
  In4/1 -> Divide2/2, Divide1/2, Divide/2

== system RPBC5602016/Single Cap2/Subsystem1 ==
  qdot : Inport
  U : Inport  Port=2
  V_c : Inport  Port=3
  Gear Ratio : Inport  Port=4
  Gain1 : Gain  Gain=1/R
  Product{,1..3} (4 alike) : Product
  Sum : Sum  Inputs=|-|+|
  alpha/R : Constant  Value=alpha/R
  Qdot : Outport
  wires:
  Product2/1 -> Sum/1
  qdot/1 -> Product3/2
  V_c/1 -> Product2/2
  Sum/1 -> Qdot/1
  alpha/R/1 -> Product1/2
  Product/1 -> Gain1/1
  U/1 -> Product/2, Product/1
  Product3/1 -> Sum/2
  Product1/1 -> Product3/1
  Gain1/1 -> Product2/1
  Gear Ratio/1 -> Product1/1

== system RPBC5602016/Single Cap2/Subsystem2 ==
  qdot : Inport
  U : Inport  Port=2
  V_c : Inport  Port=3
  Gear Ratio : Inport  Port=4
  Gain1 : Gain  Gain=1/R
  Product{,1..3} (4 alike) : Product
  Sum : Sum  Inputs=|-|+|
  alpha/R : Constant  Value=alpha/R
  Qdot : Outport
  wires:
  Gear Ratio/1 -> Product1/1
  Gain1/1 -> Product2/1
  Product1/1 -> Product3/1
  Product3/1 -> Sum/2
  U/1 -> Product/1, Product/2
  Product/1 -> Gain1/1
  alpha/R/1 -> Product1/2
  Sum/1 -> Qdot/1
  V_c/1 -> Product2/2
  qdot/1 -> Product3/2
  Product2/1 -> Sum/1

== system RPBC5602016/Single Cap2/Subsystem3 ==
  qdot : Inport
  U : Inport  Port=2
  V_c : Inport  Port=3
  Gear Ratio : Inport  Port=4
  Gain1 : Gain  Gain=1/R
  Product{,1..3} (4 alike) : Product
  Sum : Sum  Inputs=|-|+|
  alpha/R : Constant  Value=alpha/R
  Qdot : Outport
  wires:
  Product2/1 -> Sum/1
  qdot/1 -> Product3/2
  V_c/1 -> Product2/2
  Sum/1 -> Qdot/1
  alpha/R/1 -> Product1/2
  Product/1 -> Gain1/1
  U/1 -> Product/2, Product/1
  Product3/1 -> Sum/2
  Product1/1 -> Product3/1
  Gain1/1 -> Product2/1
  Gear Ratio/1 -> Product1/1

== system RPBC5602016/Single Cap3/Subsystem ==
  In1 : Inport
  In2 : Inport  Port=2
  In3 : Inport  Port=3
  In4 : Inport  Port=4
  Divide : Product  Inputs=*/
  Divide1 : Product  Inputs=*/
  Divide2 : Product  Inputs=*/
  U1 : Outport
  U2 : Outport  Port=2
  U3 : Outport  Port=3
  wires:
  In4/1 -> Divide/2, Divide1/2, Divide2/2
  In3/1 -> Divide2/1
  In2/1 -> Divide1/1
  In1/1 -> Divide/1
  Divide/1 -> U1/1
  Divide1/1 -> U2/1
  Divide2/1 -> U3/1

== system RPBC5602016/Single Cap3/Subsystem1 ==
  qdot : Inport
  U : Inport  Port=2
  V_c : Inport  Port=3
  Gear Ratio : Inport  Port=4
  Gain1 : Gain  Gain=1/R
  Product{,1..3} (4 alike) : Product
  Sum : Sum  Inputs=|-|+|
  alpha/R : Constant  Value=alpha/R
  Qdot : Outport
  wires:
  Gear Ratio/1 -> Product1/1
  Gain1/1 -> Product2/1
  Product1/1 -> Product3/1
  Product3/1 -> Sum/2
  U/1 -> Product/1, Product/2
  Product/1 -> Gain1/1
  alpha/R/1 -> Product1/2
  Sum/1 -> Qdot/1
  V_c/1 -> Product2/2
  qdot/1 -> Product3/2
  Product2/1 -> Sum/1

== system RPBC5602016/Single Cap3/Subsystem2 ==
  qdot : Inport
  U : Inport  Port=2
  V_c : Inport  Port=3
  Gear Ratio : Inport  Port=4
  Gain1 : Gain  Gain=1/R
  Product{,1..3} (4 alike) : Product
  Sum : Sum  Inputs=|-|+|
  alpha/R : Constant  Value=alpha/R
  Qdot : Outport
  wires:
  Product2/1 -> Sum/1
  qdot/1 -> Product3/2
  V_c/1 -> Product2/2
  Sum/1 -> Qdot/1
  alpha/R/1 -> Product1/2
  Product/1 -> Gain1/1
  U/1 -> Product/2, Product/1
  Product3/1 -> Sum/2
  Product1/1 -> Product3/1
  Gain1/1 -> Product2/1
  Gear Ratio/1 -> Product1/1

== system RPBC5602016/Single Cap3/Subsystem3 ==
  qdot : Inport
  U : Inport  Port=2
  V_c : Inport  Port=3
  Gear Ratio : Inport  Port=4
  Gain1 : Gain  Gain=1/R
  Product{,1..3} (4 alike) : Product
  Sum : Sum  Inputs=|-|+|
  alpha/R : Constant  Value=alpha/R
  Qdot : Outport
  wires:
  Gear Ratio/1 -> Product1/1
  Gain1/1 -> Product2/1
  Product1/1 -> Product3/1
  Product3/1 -> Sum/2
  U/1 -> Product/1, Product/2
  Product/1 -> Gain1/1
  alpha/R/1 -> Product1/2
  Sum/1 -> Qdot/1
  V_c/1 -> Product2/2
  qdot/1 -> Product3/2
  Product2/1 -> Sum/1

== system RPBC5602016/Single Cap4/Subsystem ==
  In1 : Inport
  In2 : Inport  Port=2
  In3 : Inport  Port=3
  In4 : Inport  Port=4
  Divide : Product  Inputs=*/
  Divide1 : Product  Inputs=*/
  Divide2 : Product  Inputs=*/
  U1 : Outport
  U2 : Outport  Port=2
  U3 : Outport  Port=3
  wires:
  Divide2/1 -> U3/1
  Divide1/1 -> U2/1
  Divide/1 -> U1/1
  In1/1 -> Divide/1
  In2/1 -> Divide1/1
  In3/1 -> Divide2/1
  In4/1 -> Divide2/2, Divide1/2, Divide/2

== system RPBC5602016/Single Cap4/Subsystem1 ==
  qdot : Inport
  U : Inport  Port=2
  V_c : Inport  Port=3
  Gear Ratio : Inport  Port=4
  Gain1 : Gain  Gain=1/R
  Product{,1..3} (4 alike) : Product
  Sum : Sum  Inputs=|-|+|
  alpha/R : Constant  Value=alpha/R
  Qdot : Outport
  wires:
  Product2/1 -> Sum/1
  qdot/1 -> Product3/2
  V_c/1 -> Product2/2
  Sum/1 -> Qdot/1
  alpha/R/1 -> Product1/2
  Product/1 -> Gain1/1
  U/1 -> Product/2, Product/1
  Product3/1 -> Sum/2
  Product1/1 -> Product3/1
  Gain1/1 -> Product2/1
  Gear Ratio/1 -> Product1/1

== system RPBC5602016/Single Cap4/Subsystem2 ==
  qdot : Inport
  U : Inport  Port=2
  V_c : Inport  Port=3
  Gear Ratio : Inport  Port=4
  Gain1 : Gain  Gain=1/R
  Product{,1..3} (4 alike) : Product
  Sum : Sum  Inputs=|-|+|
  alpha/R : Constant  Value=alpha/R
  Qdot : Outport
  wires:
  Gear Ratio/1 -> Product1/1
  Gain1/1 -> Product2/1
  Product1/1 -> Product3/1
  Product3/1 -> Sum/2
  U/1 -> Product/1, Product/2
  Product/1 -> Gain1/1
  alpha/R/1 -> Product1/2
  Sum/1 -> Qdot/1
  V_c/1 -> Product2/2
  qdot/1 -> Product3/2
  Product2/1 -> Sum/1

== system RPBC5602016/Single Cap4/Subsystem3 ==
  qdot : Inport
  U : Inport  Port=2
  V_c : Inport  Port=3
  Gear Ratio : Inport  Port=4
  Gain1 : Gain  Gain=1/R
  Product{,1..3} (4 alike) : Product
  Sum : Sum  Inputs=|-|+|
  alpha/R : Constant  Value=alpha/R
  Qdot : Outport
  wires:
  Product2/1 -> Sum/1
  qdot/1 -> Product3/2
  V_c/1 -> Product2/2
  Sum/1 -> Qdot/1
  alpha/R/1 -> Product1/2
  Product/1 -> Gain1/1
  U/1 -> Product/2, Product/1
  Product3/1 -> Sum/2
  Product1/1 -> Product3/1
  Gain1/1 -> Product2/1
  Gear Ratio/1 -> Product1/1

== system RPBC5602016/Single Cap5/Subsystem ==
  In1 : Inport
  In2 : Inport  Port=2
  In3 : Inport  Port=3
  In4 : Inport  Port=4
  Divide : Product  Inputs=*/
  Divide1 : Product  Inputs=*/
  Divide2 : Product  Inputs=*/
  U1 : Outport
  U2 : Outport  Port=2
  U3 : Outport  Port=3
  wires:
  In4/1 -> Divide/2, Divide1/2, Divide2/2
  In3/1 -> Divide2/1
  In2/1 -> Divide1/1
  In1/1 -> Divide/1
  Divide/1 -> U1/1
  Divide1/1 -> U2/1
  Divide2/1 -> U3/1

== system RPBC5602016/Single Cap5/Subsystem1 ==
  qdot : Inport
  U : Inport  Port=2
  V_c : Inport  Port=3
  Gear Ratio : Inport  Port=4
  Gain1 : Gain  Gain=1/R
  Product{,1..3} (4 alike) : Product
  Sum : Sum  Inputs=|-|+|
  alpha/R : Constant  Value=alpha/R
  Qdot : Outport
  wires:
  Gear Ratio/1 -> Product1/1
  Gain1/1 -> Product2/1
  Product1/1 -> Product3/1
  Product3/1 -> Sum/2
  U/1 -> Product/1, Product/2
  Product/1 -> Gain1/1
  alpha/R/1 -> Product1/2
  Sum/1 -> Qdot/1
  V_c/1 -> Product2/2
  qdot/1 -> Product3/2
  Product2/1 -> Sum/1

== system RPBC5602016/Single Cap5/Subsystem2 ==
  qdot : Inport
  U : Inport  Port=2
  V_c : Inport  Port=3
  Gear Ratio : Inport  Port=4
  Gain1 : Gain  Gain=1/R
  Product{,1..3} (4 alike) : Product
  Sum : Sum  Inputs=|-|+|
  alpha/R : Constant  Value=alpha/R
  Qdot : Outport
  wires:
  Product2/1 -> Sum/1
  qdot/1 -> Product3/2
  V_c/1 -> Product2/2
  Sum/1 -> Qdot/1
  alpha/R/1 -> Product1/2
  Product/1 -> Gain1/1
  U/1 -> Product/2, Product/1
  Product3/1 -> Sum/2
  Product1/1 -> Product3/1
  Gain1/1 -> Product2/1
  Gear Ratio/1 -> Product1/1

== system RPBC5602016/Single Cap5/Subsystem3 ==
  qdot : Inport
  U : Inport  Port=2
  V_c : Inport  Port=3
  Gear Ratio : Inport  Port=4
  Gain1 : Gain  Gain=1/R
  Product{,1..3} (4 alike) : Product
  Sum : Sum  Inputs=|-|+|
  alpha/R : Constant  Value=alpha/R
  Qdot : Outport
  wires:
  Gear Ratio/1 -> Product1/1
  Gain1/1 -> Product2/1
  Product1/1 -> Product3/1
  Product3/1 -> Sum/2
  U/1 -> Product/1, Product/2
  Product/1 -> Gain1/1
  alpha/R/1 -> Product1/2
  Sum/1 -> Qdot/1
  V_c/1 -> Product2/2
  qdot/1 -> Product3/2
  Product2/1 -> Sum/1

== system RPBC5602016/Single Cap6/Subsystem ==
  In1 : Inport
  In2 : Inport  Port=2
  In3 : Inport  Port=3
  In4 : Inport  Port=4
  Divide : Product  Inputs=*/
  Divide1 : Product  Inputs=*/
  Divide2 : Product  Inputs=*/
  U1 : Outport
  U2 : Outport  Port=2
  U3 : Outport  Port=3
  wires:
  Divide2/1 -> U3/1
  Divide1/1 -> U2/1
  Divide/1 -> U1/1
  In1/1 -> Divide/1
  In2/1 -> Divide1/1
  In3/1 -> Divide2/1
  In4/1 -> Divide2/2, Divide1/2, Divide/2

== system RPBC5602016/Single Cap6/Subsystem1 ==
  qdot : Inport
  U : Inport  Port=2
  V_c : Inport  Port=3
  Gear Ratio : Inport  Port=4
  Gain1 : Gain  Gain=1/R
  Product{,1..3} (4 alike) : Product
  Sum : Sum  Inputs=|-|+|
  alpha/R : Constant  Value=alpha/R
  Qdot : Outport
  wires:
  Product2/1 -> Sum/1
  qdot/1 -> Product3/2
  V_c/1 -> Product2/2
  Sum/1 -> Qdot/1
  alpha/R/1 -> Product1/2
  Product/1 -> Gain1/1
  U/1 -> Product/2, Product/1
  Product3/1 -> Sum/2
  Product1/1 -> Product3/1
  Gain1/1 -> Product2/1
  Gear Ratio/1 -> Product1/1

== system RPBC5602016/Single Cap6/Subsystem2 ==
  qdot : Inport
  U : Inport  Port=2
  V_c : Inport  Port=3
  Gear Ratio : Inport  Port=4
  Gain1 : Gain  Gain=1/R
  Product{,1..3} (4 alike) : Product
  Sum : Sum  Inputs=|-|+|
  alpha/R : Constant  Value=alpha/R
  Qdot : Outport
  wires:
  Gear Ratio/1 -> Product1/1
  Gain1/1 -> Product2/1
  Product1/1 -> Product3/1
  Product3/1 -> Sum/2
  U/1 -> Product/1, Product/2
  Product/1 -> Gain1/1
  alpha/R/1 -> Product1/2
  Sum/1 -> Qdot/1
  V_c/1 -> Product2/2
  qdot/1 -> Product3/2
  Product2/1 -> Sum/1

== system RPBC5602016/Single Cap6/Subsystem3 ==
  qdot : Inport
  U : Inport  Port=2
  V_c : Inport  Port=3
  Gear Ratio : Inport  Port=4
  Gain1 : Gain  Gain=1/R
  Product{,1..3} (4 alike) : Product
  Sum : Sum  Inputs=|-|+|
  alpha/R : Constant  Value=alpha/R
  Qdot : Outport
  wires:
  Product2/1 -> Sum/1
  qdot/1 -> Product3/2
  V_c/1 -> Product2/2
  Sum/1 -> Qdot/1
  alpha/R/1 -> Product1/2
  Product/1 -> Gain1/1
  U/1 -> Product/2, Product/1
  Product3/1 -> Sum/2
  Product1/1 -> Product3/1
  Gain1/1 -> Product2/1
  Gear Ratio/1 -> Product1/1

== system RPBC5602016/Single Cap7/Subsystem ==
  In1 : Inport
  In2 : Inport  Port=2
  In3 : Inport  Port=3
  In4 : Inport  Port=4
  Divide : Product  Inputs=*/
  Divide1 : Product  Inputs=*/
  Divide2 : Product  Inputs=*/
  U1 : Outport
  U2 : Outport  Port=2
  U3 : Outport  Port=3
  wires:
  Divide2/1 -> U3/1
  Divide1/1 -> U2/1
  Divide/1 -> U1/1
  In1/1 -> Divide/1
  In2/1 -> Divide1/1
  In3/1 -> Divide2/1
  In4/1 -> Divide2/2, Divide1/2, Divide/2

== system RPBC5602016/Single Cap7/Subsystem1 ==
  qdot : Inport
  U : Inport  Port=2
  V_c : Inport  Port=3
  Gear Ratio : Inport  Port=4
  Gain1 : Gain  Gain=1/R
  Product{,1..3} (4 alike) : Product
  Sum : Sum  Inputs=|-|+|
  alpha/R : Constant  Value=alpha/R
  Qdot : Outport
  wires:
  Product2/1 -> Sum/1
  qdot/1 -> Product3/2
  V_c/1 -> Product2/2
  Sum/1 -> Qdot/1
  alpha/R/1 -> Product1/2
  Product/1 -> Gain1/1
  U/1 -> Product/2, Product/1
  Product3/1 -> Sum/2
  Product1/1 -> Product3/1
  Gain1/1 -> Product2/1
  Gear Ratio/1 -> Product1/1

== system RPBC5602016/Single Cap7/Subsystem2 ==
  qdot : Inport
  U : Inport  Port=2
  V_c : Inport  Port=3
  Gear Ratio : Inport  Port=4
  Gain1 : Gain  Gain=1/R
  Product{,1..3} (4 alike) : Product
  Sum : Sum  Inputs=|-|+|
  alpha/R : Constant  Value=alpha/R
  Qdot : Outport
  wires:
  Gear Ratio/1 -> Product1/1
  Gain1/1 -> Product2/1
  Product1/1 -> Product3/1
  Product3/1 -> Sum/2
  U/1 -> Product/1, Product/2
  Product/1 -> Gain1/1
  alpha/R/1 -> Product1/2
  Sum/1 -> Qdot/1
  V_c/1 -> Product2/2
  qdot/1 -> Product3/2
  Product2/1 -> Sum/1

== system RPBC5602016/Single Cap7/Subsystem3 ==
  qdot : Inport
  U : Inport  Port=2
  V_c : Inport  Port=3
  Gear Ratio : Inport  Port=4
  Gain1 : Gain  Gain=1/R
  Product{,1..3} (4 alike) : Product
  Sum : Sum  Inputs=|-|+|
  alpha/R : Constant  Value=alpha/R
  Qdot : Outport
  wires:
  Product2/1 -> Sum/1
  qdot/1 -> Product3/2
  V_c/1 -> Product2/2
  Sum/1 -> Qdot/1
  alpha/R/1 -> Product1/2
  Product/1 -> Gain1/1
  U/1 -> Product/2, Product/1
  Product3/1 -> Sum/2
  Product1/1 -> Product3/1
  Gain1/1 -> Product2/1
  Gear Ratio/1 -> Product1/1

== matlab function RPBC5602016/MATLAB Function ==
  data: z input; u output; zd input; L input; K input
function u=RPBCpuma(z,zd,L,K)
%Robust passivity-based controller for the first 3 links of the PUMA 560

q1=z(1);
q2=z(2);
q3=z(3);
q1dot=z(4);
q2dot=z(5);
q3dot=z(6);

q1d=zd(1);
q2d=zd(2);
q3d=zd(3);
q1ddot=zd(4);
q2ddot=zd(5);
q3ddot=zd(6);
q1dddot=zd(7);
q2dddot=zd(8);
q3dddot=zd(9);

qtilde=[q1-q1d;q2-q2d;q3-q3d];
qtildedot=[q1dot-q1ddot;q2dot-q2ddot;q3dot-q3ddot];

%Gains
L=diag(L);
K=diag(K);
v=[q1ddot;q2ddot;q3ddot]-L*qtilde;
a=[q1dddot;q2dddot;q3dddot]-L*qtildedot;
r=qtildedot+L*qtilde;

a_1=a(1);a_2=a(2);a_3=a(3);
v_1=v(1);v_2=v(2);v_3=v(3);
B_e=[38.7871 114.0474 28.5225];
%Form the regressor
Yav1=[a_1, a_1*cos(q2)^2 - q1dot*v_2*cos(q2)*sin(q2) - q2dot*v_1*cos(q2)*sin(q2), a_1*cos(q2 + q3)^2 - v_1*(q2dot*cos(q2 + q3)*sin(q2 + q3) + q3dot*cos(q2 + q3)*sin(q2 + q3)) - q1dot*v_2*cos(q2 + q3)*sin(q2 + q3) - q1dot*v_3*cos(q2 + q3)*sin(q2 + q3), 2*a_1*cos(q2 + q3)*cos(q2) - v_1*(q2dot*(cos(q2 + q3)*sin(q2) + sin(q2 + q3)*cos(q2)) + q3dot*sin(q2 + q3)*cos(q2)) - q1dot*v_2*(cos(q2 + q3)*sin(q2) + sin(q2 + q3)*cos(q2)) - q1dot*v_3*sin(q2 + q3)*cos(q2), v_2*(q2dot*cos(q2 + q3) + q3dot*cos(q2 + q3)) + v_3*(q2dot*cos(q2 + q3) + q3dot*cos(q2 + q3)) + a_2*sin(q2 + q3) + a_3*sin(q2 + q3), 0, 0, a_2*sin(q2) + q2dot*v_2*cos(q2), 0, 0,B_e(1)*q1dot];
Yav2=[ 0, q1dot*v_1*cos(q2)*sin(q2), q1dot*v_1*cos(q2 + q3)*sin(q2 + q3), 2*a_2*cos(q3) + a_3*cos(q3) - v_3*(q2dot*sin(q3) + q3dot*sin(q3)) - q3dot*v_2*sin(q3) + q1dot*v_1*(cos(q2 + q3)*sin(q2) + sin(q2 + q3)*cos(q2)), a_1*sin(q2 + q3), a_2, a_3, a_1*sin(q2), -cos(q2 + q3), -cos(q2),B_e(2*q2dot)];
Yav3=[ 0, 0, q1dot*v_1*cos(q2 + q3)*sin(q2 + q3), a_2*cos(q3) + q2dot*v_2*sin(q3) + q1dot*v_1*sin(q2 + q3)*cos(q2), a_1*sin(q2 + q3), 0, a_2 + a_3, 0, -cos(q2 + q3), 0,B_e(3)*q3dot];

Yav=[Yav1;Yav2;Yav3];
%Nominal parameters 
TH0 =[
    2.8123
    2.2623
    -0.0066
    0.3453
   -0.08499
    8.8038
    1.0711
   -0.9748
    6.8067
   55.35
        1];
   
deadzone=0.2;
rho=32;
s=Yav'*r;
if norm(s)>deadzone
    dTh=-rho*s/norm(s);
else
    dTh=-rho*s/deadzone;
end
Th_hat=TH0+dTh;
%Effective input constant inverse (Volts/(Nm))
Kui=diag([0.1223 0.0713 0.1426]);
T=Yav*Th_hat-K*r;
u=Kui*(T);
